simulink model "ee_motor_pmsm_drive"  (R2020b)
settings: Solver=ode23t  StartTime=0.0  StopTime=0.377  MaxStep=1e-6  RelTol=1e-4  AbsTol=1e-3  EnableMultiTasking=on
PreLoadFcn:
  | tsim = 0.05;
PostLoadFcn:
  | % Create the PMSM data
  | ee_motor_pmsm_drive_params
  | 
  | % Test harness test point
  | rpm0 = 1400;
  | torque0 = 200;
InitFcn:
  | % Set simulation time for 5 full AC cycles
  | tsim = 5*60/rpm0/N;
StopFcn:
  | ee_addSimlogTimeStamp(bdroot)
undefined symbols (not defined in the file): N, Ts
libraries: fl_lib x10, nesl_utility x7, ee_lib x1
CloseFcn:
  | try,close(h1_ee_motor_pmsm_drive),end
  | clear h1_ee_motor_pmsm_drive
  | try,close(h2_ee_motor_pmsm_drive),end
  | clear h2_ee_motor_pmsm_drive
  | try,close(h3_ee_motor_pmsm_drive),end
  | clear h3_ee_motor_pmsm_drive
  | try,close(h4_ee_motor_pmsm_drive),end
  | clear h4_ee_motor_pmsm_drive
  | 
  | 
  | clear simlog_ee_motor_pmsm_drive
  | clear logsout_ee_motor_pmsm_drive
  | clear Imax L0 Ld Lq N PM Pmax Rs Tmax TorqueMatrix Ts Tsc dfluxAdiaMatrix dfluxAdibMatrix dfluxAdicMatrix dfluxAdxMatrix efficiency fc fnom fsw iDC idVec iqVec omegam_nom powerDC powerLosses rpm0 rpm_nom t tMax tMin tabulatedLosses time torque0 totalLosses tout tsim vDC xVec
Description:
  | HEV PMSM Drive Test Harness
settings Model: Creator=The MathWorks, Inc.  LastModifiedBy=ge62gas
settings SolverCC: AutoScaleAbsTol=off  MaxConsecutiveMinStep=2
settings DataIOCC: LimitDataPoints=on  MaxDataPoints=35000  SaveFormat=StructureWithTime  SaveOutput=off  DSMLogging=off  ReturnWorkspaceOutputs=off  SignalLoggingName=logsout_ee_motor_pmsm_drive
settings OptimizationCC: LifeSpan=inf
settings DebuggingCC: UnderspecifiedInitializationDetection=Classic  MergeDetectMultiDrivingBlocksExec=none  AllowSymbolicDim=off  PregeneratedLibrarySubsystemCodeDiagnostic=none  SFUnexpectedBacktrackingDiag=warning  SFNoUnconditionalDefaultTransitionDiag=warning  SFExecutionAtInitializationDiag=none  ArithmeticOperatorsInVariantConditions=warning
settings HardwareCC: ProdBitPerPointer=32  ProdBitPerSizeT=32  ProdBitPerPtrDiffT=32  ProdLargestAtomicFloat=None  ProdIntDivRoundTo=Undefined  ProdEndianess=Unspecified  ProdWordSize=32  ProdHWDeviceType=32-bit Generic
settings ModelReferenceCC: PropagateSignalLabelsOutOfModel=off
settings SFSimCC: SimUseLocalCustomCode=off
settings RTWCC: RTWUseLocalCustomCode=off
settings CodeAppCC: StateflowObjectComments=on
settings GRTTargetCC: TargetLangStandard=C89/C90 (ANSI)
settings ConfigComp: CovMetricSettings=dw  CovSaveCumulativeToWorkspaceVar=on  CovSaveSingleToWorkspaceVar=on  CovExternalEMLEnable=off  CovSFcnEnable=off
settings SimscapeCC: SimscapeLogType=all  SimscapeLogSimulationStatistics=on  SimscapeLogName=simlog_ee_motor_pmsm_drive  SimscapeLogDecimation=10  SimscapeLogDataHistory=1000000

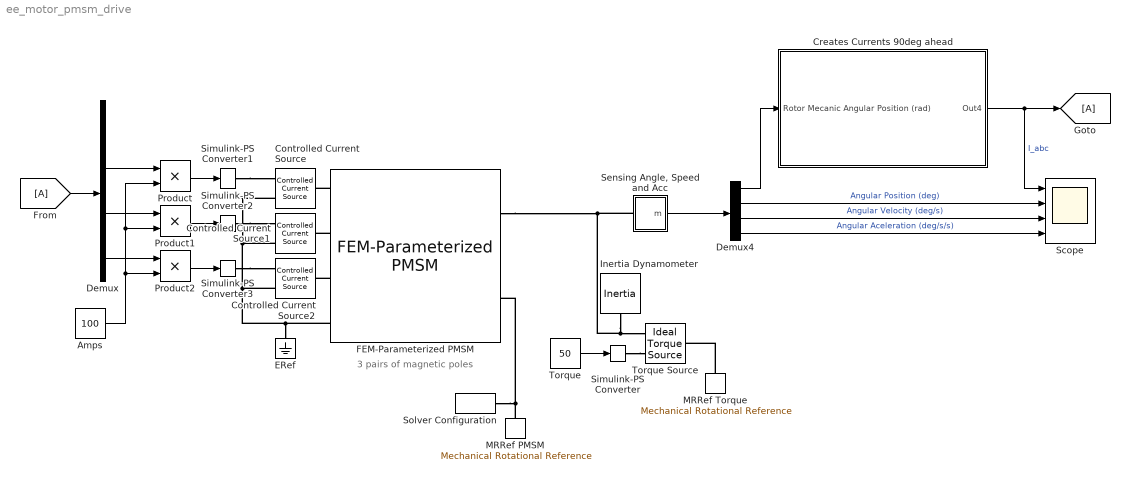
== system ee_motor_pmsm_drive ==
  note: 3 pairs of magnetic poles
  Amps : Constant  Value=100
  Controlled Current Source : fl_lib/Electrical/Electrical Sources/Controlled Current Source
  Controlled Current Source1 : fl_lib/Electrical/Electrical Sources/Controlled Current Source
  Controlled Current Source2 : fl_lib/Electrical/Electrical Sources/Controlled Current Source
  Creates Currents 90deg ahead : Subsystem
  Demux : Demux
  Demux4 : Demux
  ERef : fl_lib/Electrical/Electrical Elements/Electrical Reference
      settings: SourceProductName=Foundation Library
  FEM-Parameterized PMSM : ee_lib/Electromechanical/Permanent Magnet/FEM-Parameterized PMSM  parameterization=1  winding_type=ee.enum.statorconnection.wye  iVec=[-2, 0, 2] A  xVec=xVec rad  dfluxdiMatrix=0.0002 * ones(3, 4) Wb/A  dfluxdxMatrix=[0, -.16, .16, 0; 0, -.16, .16, 0; 0, -.16, .16, 0] Wb/rad  calculate_torque_matrix=1  TorqueMatrix=zeros(3, 3, 3, 4) N*m  idVec1=[-200, 0, 200] A  iqVec1=[-200, 0, 200] A  LdMatrix=0.0002 * ones(3, 3) H  LqMatrix=0.0002 * ones(3, 3) H  PmMatrix=0.1 * ones(3, 3) Wb  N=6  interp_method=simscape.enum.interpolation.smooth  Rs=Rs Ohm  Ms=0.00002 H  L0=0.00016 H  losses_oc=[500 1500 0] W  losses_sc=[200 600 0] W  f_losses=140 Hz  Isc_losses=350 A  Inertia=0.01 kg*m^2  lam=0 N*m/(rad/s)  i_d_specify=off  i_d_priority=High  i_d=0 A  i_d_nominal_specify=off  i_d_nominal_unit=A  i_d_nominal_value=1  i_q_specify=off  i_q_priority=High  i_q=0 A  i_q_nominal_specify=off  i_q_nominal_unit=A  i_q_nominal_value=1  torque_specify=off  torque_priority=None  torque=0 N*m  torque_nominal_specify=off  torque_nominal_unit=N*m  torque_nominal_value=1  angular_velocity_specify=off  angular_velocity_priority=High  angular_velocity=0 deg/s  angular_velocity_nominal_specify=off  angular_velocity_nominal_unit=rpm  angular_velocity_nominal_value=1  angular_position_specify=on  angular_position_priority=High  angular_position=0 rad  angular_position_nominal_specify=off  angular_position_nominal_unit=deg  angular_position_nominal_value=1  Tmeas=298.15 K  alpha=3.93e-3 1/K  alpha_flux=-0.001 1/K  stator_thermal_mass=100 J/K  stator_initial_temperatures=[298.15, 298.15, 298.15] K  rotor_thermal_mass=200 J/K  rotor_initial_temperature=298.15 K  Rm_percent_rotor=90  Rd_percent_rotor=30  idVec=idVec A  iqVec=iqVec A  dfluxAdiaMatrix3D=dfluxAdiaMatrix Wb/A  dfluxAdibMatrix3D=dfluxAdibMatrix Wb/A  dfluxAdicMatrix3D=dfluxAdicMatrix Wb/A  dfluxAdxMatrix3D=dfluxAdxMatrix Wb/rad  TorqueMatrix3D=TorqueMatrix N*m  iaVec=[-200, 0, 200] A  ibVec=[-200, 0, 200] A  icVec=[-200, 0, 200] A  dfluxAdiaMatrix=zeros(3, 3, 3, 4) Wb/A  dfluxAdibMatrix=zeros(3, 3, 3, 4) Wb/A  dfluxAdicMatrix=zeros(3, 3, 3, 4) Wb/A  dfluxAdxMatrix=zeros(3, 3, 3, 4) Wb/rad  param_dq0=1  winding_type_dq0=1  nPolePairs=4  parks_type=1  idVec2=[-200, 0, 200] A  iqVec2=[-200, 0, 200] A  magVec2=[0, 100, 200] A  betaVec2=[-180, -90, 0, 90, 180] deg  xVec2=[0, 5, 10, 15, 20, 25, 30] deg  fluxD_dq0=zeros(3, 3, 7) Wb  fluxQ_dq0=zeros(3, 3, 7) Wb  fluxA_dq0=zeros(3, 3, 7) Wb  Torque_dq0=zeros(3, 3, 7) N*m  fluxD_IBX=zeros(3, 5, 7) Wb  fluxQ_IBX=zeros(3, 5, 7) Wb  fluxA_IBX=zeros(3, 5, 7) Wb  Torque_IBX=zeros(3, 5, 7) N*m
      settings: SourceProductName=Electrical  LogSimulationData=on  InternalSimscapePortConfiguration="{\"Bottom\":[],\"Left\":[{\"id\":\"a\",\"label\":\"a\",\"type\":\"foundation.electrical.electrical\"},{\"id\":\"b\",\"label\":\"b\",\"type\":\"foundation.electrical.electrical\"},{\"id\":\"c\",\"label\":\"c\",\"type\":\"foundation.electrical.electrical\"},{\"id\":\"n\",\"label\":\"n\",\"type\":\"foundation.electrical.electrical\"}],\"Right\":[{\"id\":\"R\",\"label\":\"R\",\"type\":\"foundation.mechanical.rotational.rotational\"},{\"id\":\"C\",\"label\":\"C\",\"type\":\"foundation.mechanical.rotational.rotational\"}],\"Top\":[]}"
  Inertia Dynamometer : fl_lib/Mechanical/Rotational Elements/Inertia  inertia=1 kg*m^2  num_ports=foundation.enum.numPorts2.one  w_specify=on  w_priority=High  w=rpm0 rpm  w_nominal_specify=off  w_nominal_unit=rad/s  w_nominal_value=1  t_specify=off  t_priority=High  t=0 N*m  t_nominal_specify=off  t_nominal_unit=N*m  t_nominal_value=1
      settings: SourceProductName=Foundation Library
  MRRef PMSM : fl_lib/Mechanical/Rotational Elements/Mechanical Rotational Reference
      settings: SourceProductName=Foundation Library
  MRRef Torque : fl_lib/Mechanical/Rotational Elements/Mechanical Rotational Reference
      settings: SourceProductName=Foundation Library
  Product : Product
  Product1 : Product
  Product2 : Product
  Scope : Scope  NumInputPorts=4
  "Sensing Angle, Speed and Acc" : Subsystem
      mask Display: disp('m')
  Simulink-PS Converter : nesl_utility/Simulink-PS Converter  PhysicalDomain=network_engine_domain  SubClassName=ps_input  LeftPortType=input  RightPortType=output  PseudoPeriodic=off  Frequencies=[]  NoiseDistribution=none  NoiseParameters=[]  Unit=1  AffineConversion=off  FilteringAndDerivatives=provide  SimscapeFilterOrder=1  InputFilterTimeConstant=0.001  UdotUserProvided=0
  Simulink-PS Converter1 : nesl_utility/Simulink-PS Converter  PhysicalDomain=network_engine_domain  SubClassName=ps_input  LeftPortType=input  RightPortType=output  PseudoPeriodic=off  Frequencies=[]  NoiseDistribution=none  NoiseParameters=[]  Unit=A  AffineConversion=off  FilteringAndDerivatives=filter  SimscapeFilterOrder=1  InputFilterTimeConstant=0.001  UdotUserProvided=0
  Simulink-PS Converter2 : nesl_utility/Simulink-PS Converter  PhysicalDomain=network_engine_domain  SubClassName=ps_input  LeftPortType=input  RightPortType=output  PseudoPeriodic=off  Frequencies=[]  NoiseDistribution=none  NoiseParameters=[]  Unit=A  AffineConversion=off  FilteringAndDerivatives=filter  SimscapeFilterOrder=1  InputFilterTimeConstant=0.001  UdotUserProvided=0
  Simulink-PS Converter3 : nesl_utility/Simulink-PS Converter  PhysicalDomain=network_engine_domain  SubClassName=ps_input  LeftPortType=input  RightPortType=output  PseudoPeriodic=off  Frequencies=[]  NoiseDistribution=none  NoiseParameters=[]  Unit=A  AffineConversion=off  FilteringAndDerivatives=filter  SimscapeFilterOrder=1  InputFilterTimeConstant=0.001  UdotUserProvided=0
  Solver Configuration : nesl_utility/Solver Configuration  PhysicalDomain=network_engine_domain  SubClassName=solver  LeftPortType=input  RightPortType=generic  Tones=[]  Harmonics=[]  SimulateNoise=off  Profile=off  UseLocalSampling=off  EnableSwitchedLinearOptims=on  FrequencyDomain=off  UseCCode=off  RelTol=0.001  AbsTol=1e-06  MinStep=1e-09  ToWorkspace=off  RevertToSquareIcSolve=off  NumHomotopyIterations=100  PhasorMode=off  PhasorModeNumHarmonics=1  DoDC=off  ResidualTolerance=1e-9  UseLocalSolver=off  LocalSolverChoice=NE_BACKWARD_EULER_ADVANCER  LocalSolverSampleTime=Ts/1000  DoFixedCost=on  MaxNonlinIter=4  MaxModeIter=2  ComputeImpulses=off  ImpulseIterations=2  LinearAlgebra=auto  EquationFormulation=NE_TIME_EF  DelaysMemoryBudget=1024  AutomaticFiltering=on  FilteringTimeConstant=0.001  PartitionStorageMethod=AS_NEEDED  PartitionMemoryBudget=1024  PartitionMethod=FAST
      settings: SourceProductName=Utilities
  Torque : Constant  Value=50
  Torque Source : fl_lib/Mechanical/Mechanical Sources/Ideal Torque Source
      settings: SourceProductName=Foundation Library
  wires:
  Demux4/2 -> Scope/2  "Angular Position (deg)"
  "Sensing Angle, Speed and Acc"/1(m) -> Demux4/1
  Torque/1 -> Simulink-PS Converter/1
  Amps/1 -> Product2/2, Product/2, Product1/2
  Product/1 -> Simulink-PS Converter1/1
  Product2/1 -> Simulink-PS Converter3/1
  Product1/1 -> Simulink-PS Converter2/1
  Demux4/3 -> Scope/3  "Angular Velocity (deg/s)"
  Demux4/4 -> Scope/4  "Angular Aceleration (deg/s/s)"
  Demux4/1 -> Creates Currents 90deg ahead/1(Rotor Mecanic Angular Position (rad))
  Creates Currents 90deg ahead/1(Out4) -> [A], Scope/1  "I_abc"
  [A] -> Demux/1
  Demux/3 -> Product1/1
  Demux/4 -> Product2/1
  Demux/2 -> Product/1
  connections:
  Inertia Dynamometer/LConn1 -- FEM-Parameterized PMSM/RConn1 -- "Sensing Angle, Speed and Acc"/LConn1 -- Torque Source/RConn2
  Controlled Current Source/RConn2 -- Controlled Current Source1/RConn2 -- FEM-Parameterized PMSM/LConn4 -- ERef/LConn1 -- Controlled Current Source2/RConn2
  MRRef PMSM/LConn1 -- FEM-Parameterized PMSM/RConn2 -- Solver Configuration/RConn1
  MRRef Torque/LConn1 -- Torque Source/LConn1
  Simulink-PS Converter/RConn1 -- Torque Source/RConn1
  FEM-Parameterized PMSM/LConn1 -- Controlled Current Source/LConn1
  Simulink-PS Converter1/RConn1 -- Controlled Current Source/RConn1
  Simulink-PS Converter2/RConn1 -- Controlled Current Source1/RConn1
  Simulink-PS Converter3/RConn1 -- Controlled Current Source2/RConn1
  FEM-Parameterized PMSM/LConn2 -- Controlled Current Source1/LConn1
  FEM-Parameterized PMSM/LConn3 -- Controlled Current Source2/LConn1

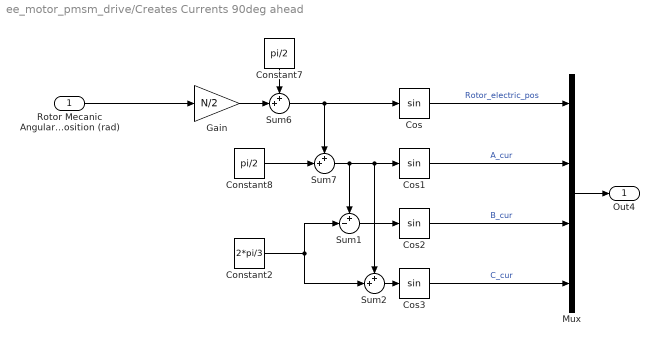
== system ee_motor_pmsm_drive/Creates Currents 90deg ahead ==
  Rotor Mecanic Angular Position (rad) : Inport
  Constant2 : Constant  Value=2*pi/3
  Constant7 : Constant  Value=pi/2
  Constant8 : Constant  Value=pi/2
  Cos{,1..3} (4 alike) : Trigonometry
  Gain : Gain  Gain=N/2
  Mux : Mux
  Sum1 : Sum  Inputs=+-|
  Sum2 : Sum  Inputs=++|
  Sum6 : Sum  Inputs=++|
  Sum7 : Sum  Inputs=++|
  Out4 : Outport
  wires:
  Sum7/1 -> Sum1/1, Sum2/1, Cos1/1
  Cos3/1 -> Mux/4  "C_cur"
  Sum2/1 -> Cos3/1
  Sum6/1 -> Cos/1, Sum7/1
  Sum1/1 -> Cos2/1
  Rotor Mecanic Angular Position (rad)/1 -> Gain/1
  Mux/1 -> Out4/1
  Constant8/1 -> Sum7/2
  Constant2/1 -> Sum2/2, Sum1/2
  Constant7/1 -> Sum6/1
  Gain/1 -> Sum6/2
  Cos2/1 -> Mux/3  "B_cur"
  Cos1/1 -> Mux/2  "A_cur"
  Cos/1 -> Mux/1  "Rotor_electric_pos"

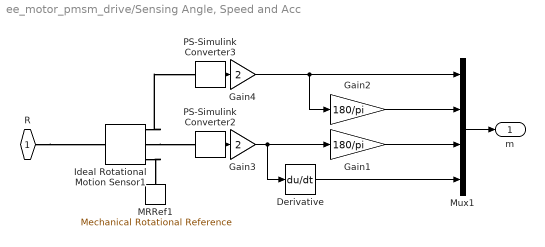
== system ee_motor_pmsm_drive/Sensing Angle, Speed and Acc ==
  Derivative : Derivative
  Gain1 : Gain  Gain=180/pi
  Gain2 : Gain  Gain=180/pi
  Gain3 : Gain  Gain=2
  Gain4 : Gain  Gain=2
  Ideal Rotational Motion Sensor1 : fl_lib/Mechanical/Mechanical Sensors/Ideal Rotational Motion Sensor  wrap_angle=simscape.enum.onoff.off  offset=0 rad
      settings: SourceProductName=Foundation Library
  MRRef1 : fl_lib/Mechanical/Rotational Elements/Mechanical Rotational Reference
      settings: SourceProductName=Foundation Library
  Mux1 : Mux
  PS-Simulink Converter2 : nesl_utility/PS-Simulink Converter  PhysicalDomain=network_engine_domain  SubClassName=ps_output  LeftPortType=input  RightPortType=output  PseudoPeriodic=off  Frequencies=[]  Unit=rad/s  AffineConversion=off
      settings: SourceProductName=Utilities
  PS-Simulink Converter3 : nesl_utility/PS-Simulink Converter  PhysicalDomain=network_engine_domain  SubClassName=ps_output  LeftPortType=input  RightPortType=output  PseudoPeriodic=off  Frequencies=[]  Unit=rad  AffineConversion=off
      settings: SourceProductName=Utilities
  R : PMIOPort  Side=Left
  m : Outport  VectorParamsAs1DForOutWhenUnconnected=off
  wires:
  Mux1/1 -> m/1
  Gain2/1 -> Mux1/2
  PS-Simulink Converter2/1 -> Gain3/1
  Gain3/1 -> Derivative/1, Gain1/1
  Gain4/1 -> Gain2/1, Mux1/1
  Gain1/1 -> Mux1/3
  PS-Simulink Converter3/1 -> Gain4/1
  Derivative/1 -> Mux1/4
  connections:
  Ideal Rotational Motion Sensor1/RConn1 -- MRRef1/LConn1
  Ideal Rotational Motion Sensor1/RConn3 -- PS-Simulink Converter3/LConn1
  Ideal Rotational Motion Sensor1/RConn2 -- PS-Simulink Converter2/LConn1
  R/RConn1 -- Ideal Rotational Motion Sensor1/LConn1
